simulink model "SMC_s"  (R2023a)
settings: Solver=VariableStepAuto  StartTime=0.0  StopTime=10.0  RelTol=1e-3
undefined symbols (not defined in the file): C_col, DiscIntNeverNeededParam, J_col, K, k_sw, lambda, Phi, tau_f, Tdref_ay_bp_ms2, Tdref_table, Tdref_v_bp_ms, Ts_ctrl
settings Model: Creator=Tan_Tram  LastModifiedBy=Tan_Tram

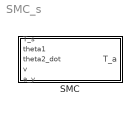
== system SMC_s ==
  SMC : Subsystem

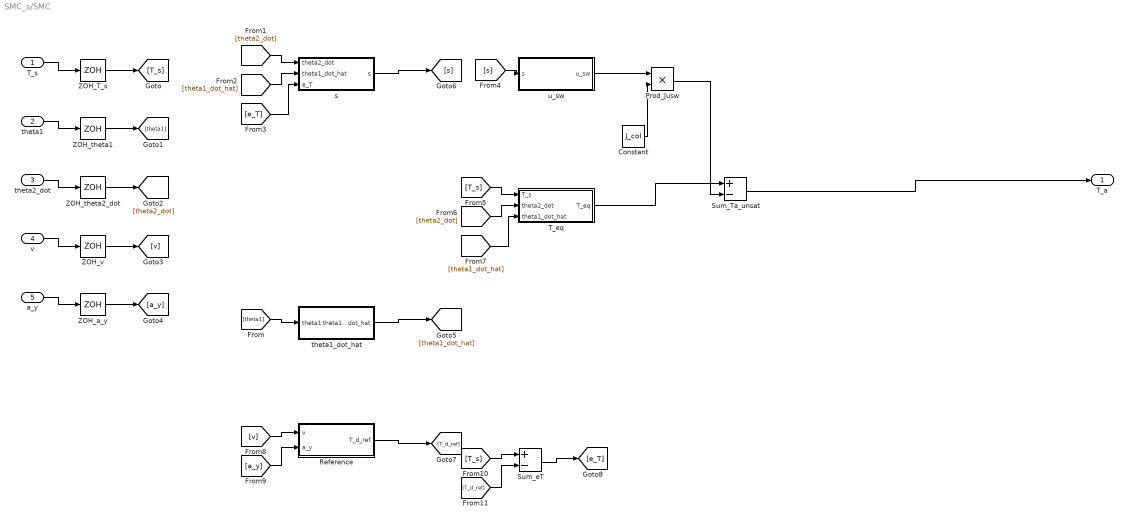
== system SMC_s/SMC ==
  T_s : Inport
  theta1 : Inport  Port=2
  theta2_dot : Inport  Port=3
  v : Inport  Port=4
  a_y : Inport  Port=5
  Constant : Constant  Value=J_col
  Prod_Jusw : Product  Inputs=**
  Reference : Subsystem
  Sum_Ta_unsat : Sum  Inputs=+-
  Sum_eT : Sum  Inputs=+-
  T_eq : Subsystem
  ZOH_T_s : ZeroOrderHold  SampleTime=Ts_ctrl
  ZOH_a_y : ZeroOrderHold  SampleTime=Ts_ctrl
  ZOH_theta1 : ZeroOrderHold  SampleTime=Ts_ctrl
  ZOH_theta2_dot : ZeroOrderHold  SampleTime=Ts_ctrl
  ZOH_v : ZeroOrderHold  SampleTime=Ts_ctrl
  s : Subsystem
  theta1_dot_hat : Subsystem
  u_sw : Subsystem
  T_a : Outport
  wires:
  T_s/1 -> ZOH_T_s/1
  ZOH_T_s/1 -> [T_s]
  theta1/1 -> ZOH_theta1/1
  ZOH_theta1/1 -> [theta1]
  theta2_dot/1 -> ZOH_theta2_dot/1
  ZOH_theta2_dot/1 -> [theta2_dot]
  v/1 -> ZOH_v/1
  ZOH_v/1 -> [v]
  a_y/1 -> ZOH_a_y/1
  ZOH_a_y/1 -> [a_y]
  [theta1] -> theta1_dot_hat/1(theta1)
  theta1_dot_hat/1(theta1_dot_hat) -> [theta1_dot_hat]
  [theta2_dot] -> s/1(theta2_dot)
  [theta1_dot_hat] -> s/2(theta1_dot_hat)
  [e_T] -> s/3(e_T)
  s/1(s) -> [s]
  [s] -> u_sw/1(s)
  [T_s] -> T_eq/1(T_s)
  [theta2_dot] -> T_eq/2(theta2_dot)
  [theta1_dot_hat] -> T_eq/3(theta1_dot_hat)
  u_sw/1(u_sw) -> Prod_Jusw/1
  Constant/1 -> Prod_Jusw/2
  T_eq/1(T_eq) -> Sum_Ta_unsat/1
  Prod_Jusw/1 -> Sum_Ta_unsat/2
  [v] -> Reference/1(v)
  [a_y] -> Reference/2(a_y)
  Reference/1(T_d_ref) -> [T_d_ref]
  [T_s] -> Sum_eT/1
  [T_d_ref] -> Sum_eT/2
  Sum_eT/1 -> [e_T]
  Sum_Ta_unsat/1 -> T_a/1

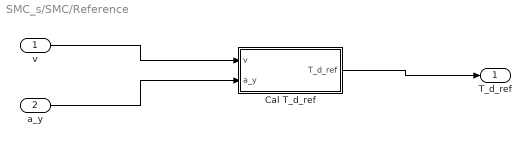
== system SMC_s/SMC/Reference ==
  v : Inport
  a_y : Inport  Port=2
  Cal T_d_ref : Subsystem
  T_d_ref : Outport
  wires:
  Cal T_d_ref/1(T_d_ref) -> T_d_ref/1
  a_y/1 -> Cal T_d_ref/2(a_y)
  v/1 -> Cal T_d_ref/1(v)

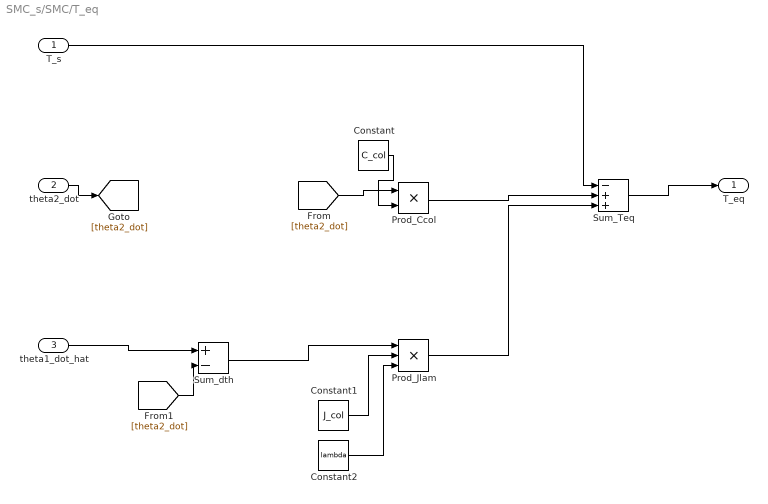
== system SMC_s/SMC/T_eq ==
  T_s : Inport
  theta2_dot : Inport  Port=2
  theta1_dot_hat : Inport  Port=3
  Constant : Constant  Value=C_col
  Constant1 : Constant  Value=J_col
  Constant2 : Constant  Value=lambda
  Prod_Ccol : Product  Inputs=**
  Prod_Jlam : Product  Inputs=***
  Sum_Teq : Sum  Inputs=-++
  Sum_dth : Sum  Inputs=+-
  T_eq : Outport
  wires:
  theta2_dot/1 -> [theta2_dot]
  [theta2_dot] -> Prod_Ccol/1
  Constant/1 -> Prod_Ccol/2
  theta1_dot_hat/1 -> Sum_dth/1
  [theta2_dot] -> Sum_dth/2
  Sum_dth/1 -> Prod_Jlam/1
  Constant1/1 -> Prod_Jlam/2
  Constant2/1 -> Prod_Jlam/3
  T_s/1 -> Sum_Teq/1
  Prod_Ccol/1 -> Sum_Teq/2
  Prod_Jlam/1 -> Sum_Teq/3
  Sum_Teq/1 -> T_eq/1

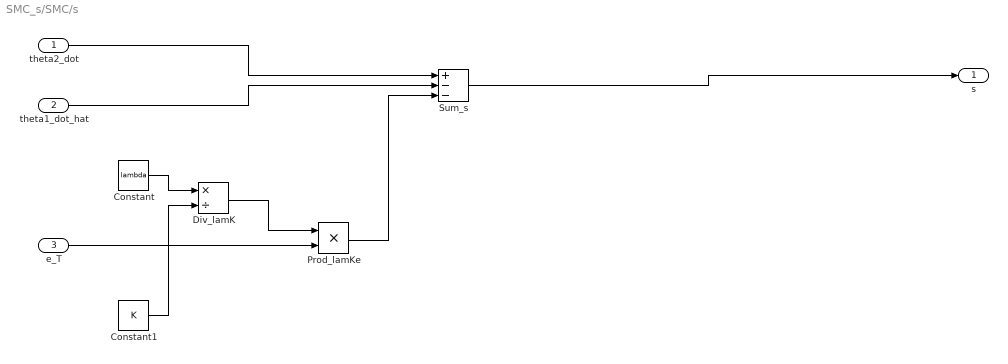
== system SMC_s/SMC/s ==
  theta2_dot : Inport
  theta1_dot_hat : Inport  Port=2
  e_T : Inport  Port=3
  Constant : Constant  Value=lambda
  Constant1 : Constant  Value=K
  Div_lamK : Product  Inputs=*/
  Prod_lamKe : Product  Inputs=**
  Sum_s : Sum  Inputs=+--
  s : Outport
  wires:
  Constant/1 -> Div_lamK/1
  Constant1/1 -> Div_lamK/2
  Div_lamK/1 -> Prod_lamKe/1
  e_T/1 -> Prod_lamKe/2
  theta2_dot/1 -> Sum_s/1
  theta1_dot_hat/1 -> Sum_s/2
  Prod_lamKe/1 -> Sum_s/3
  Sum_s/1 -> s/1

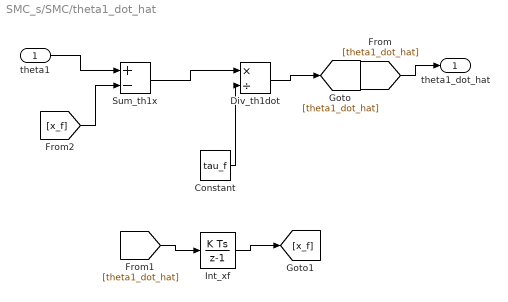
== system SMC_s/SMC/theta1_dot_hat ==
  theta1 : Inport
  Constant : Constant  Value=tau_f
  Div_th1dot : Product  Inputs=*/
  Int_xf : DiscreteIntegrator  SampleTime=Ts_ctrl  ICPrevOutput=DiscIntNeverNeededParam  ICPrevScaledInput=DiscIntNeverNeededParam
  Sum_th1x : Sum  Inputs=+-
  theta1_dot_hat : Outport
  wires:
  theta1/1 -> Sum_th1x/1
  [x_f] -> Sum_th1x/2
  Sum_th1x/1 -> Div_th1dot/1
  Constant/1 -> Div_th1dot/2
  Div_th1dot/1 -> [theta1_dot_hat]
  [theta1_dot_hat] -> theta1_dot_hat/1
  [theta1_dot_hat] -> Int_xf/1
  Int_xf/1 -> [x_f]

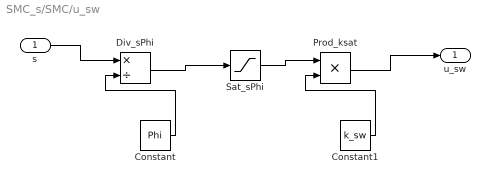
== system SMC_s/SMC/u_sw ==
  s : Inport
  Constant : Constant  Value=Phi
  Constant1 : Constant  Value=k_sw
  Div_sPhi : Product  Inputs=*/
  Prod_ksat : Product  Inputs=**
  Sat_sPhi : Saturate  UpperLimit=1  LowerLimit=-1
  u_sw : Outport
  wires:
  s/1 -> Div_sPhi/1
  Constant/1 -> Div_sPhi/2
  Div_sPhi/1 -> Sat_sPhi/1
  Sat_sPhi/1 -> Prod_ksat/1
  Constant1/1 -> Prod_ksat/2
  Prod_ksat/1 -> u_sw/1

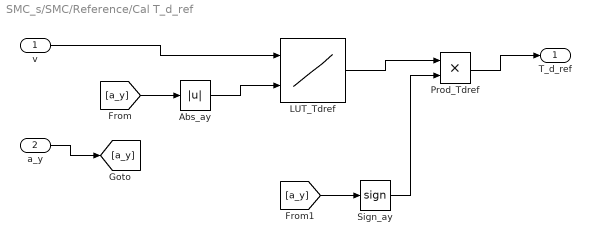
== system SMC_s/SMC/Reference/Cal T_d_ref ==
  v : Inport
  a_y : Inport  Port=2
  Abs_ay : Abs  SaturateOnIntegerOverflow=off
  LUT_Tdref : Lookup_n-D  BreakpointsForDimension1=Tdref_v_bp_ms  BreakpointsForDimension2=Tdref_ay_bp_ms2  Table=Tdref_table  ExtrapMethod=Clip  InternalRulePriority=Speed  RndMeth=Simplest
      settings: InputPortMap=u0,u1
  Prod_Tdref : Product  Inputs=**
  Sign_ay : Signum
  T_d_ref : Outport
  wires:
  Prod_Tdref/1 -> T_d_ref/1
  Sign_ay/1 -> Prod_Tdref/2
  LUT_Tdref/1 -> Prod_Tdref/1
  [a_y] -> Sign_ay/1
  Abs_ay/1 -> LUT_Tdref/2
  [a_y] -> Abs_ay/1
  v/1 -> LUT_Tdref/1
  a_y/1 -> [a_y]
